simulink model "torqueBalancingYoga2017a"  (Simulink 8.9)
settings: Solver=FixedStepDiscrete  StartTime=0.0  StopTime="Config.SIMULATION_TIME "  FixedStep=Config.Ts  RelTol=1e-3  EnableMultiTasking=on
InitFcn:
  | cd(fileparts(which(bdroot)));
  | initTorqueBalancingYoga;
StopFcn:
  | cd(fileparts(which(bdroot)));
  | stopTorqueBalancingYoga;
undefined symbols (not defined in the file or in its folder): bVectorConstraints, Config, ConstraintsMatrix, Gain, Reg, ROBOT_DOF, ROBOT_DOF_FOR_SIMULINK, Sat, Sm
libraries: WBToolboxLibrary x86, simulink x4
(part 2 of 2)

== system torqueBalancingYoga2017a/controller_QP/Compute angular momentum integral/Compute base to fixed link transform ==
  qj : Inport
  inertial : Inport  Port=2
  Constant7 : Constant  Value=eye(4)
  "LFoot to base link transform " : Subsystem
  LFoot to world transform (fixed base) : WBToolboxLibrary/wholeBodyModel/Kinematics/Forward Kinematics  frameName=Frames.LEFT_FOOT
      settings: SourceProductName=Whole Body Toolbox
  RFoot to base link transform : Subsystem
  RFoot to world transform (fixed base) : WBToolboxLibrary/wholeBodyModel/Kinematics/Forward Kinematics  frameName=Frames.RIGHT_FOOT
      settings: SourceProductName=Whole Body Toolbox
  fixed_LFoot_H_b : Outport
  fixed_RFoot_H_b : Outport  Port=2
  wires:
  Constant7/1 -> RFoot to base link transform/4(w_H_base_fixed), "LFoot to base link transform "/4(w_H_base_fixed), RFoot to world transform (fixed base)/1, LFoot to world transform (fixed base)/1
  RFoot to base link transform/1(link_H_b) -> fixed_RFoot_H_b/1
  "LFoot to base link transform "/1(link_H_b) -> fixed_LFoot_H_b/1
  LFoot to world transform (fixed base)/1 -> "LFoot to base link transform "/3(w_H_link)
  RFoot to world transform (fixed base)/1 -> RFoot to base link transform/3(w_H_link)
  qj/1 -> "LFoot to base link transform "/1(qj), RFoot to base link transform/1(qj), RFoot to world transform (fixed base)/2, LFoot to world transform (fixed base)/2
  inertial/1 -> "LFoot to base link transform "/2(inertial), RFoot to base link transform/2(inertial)

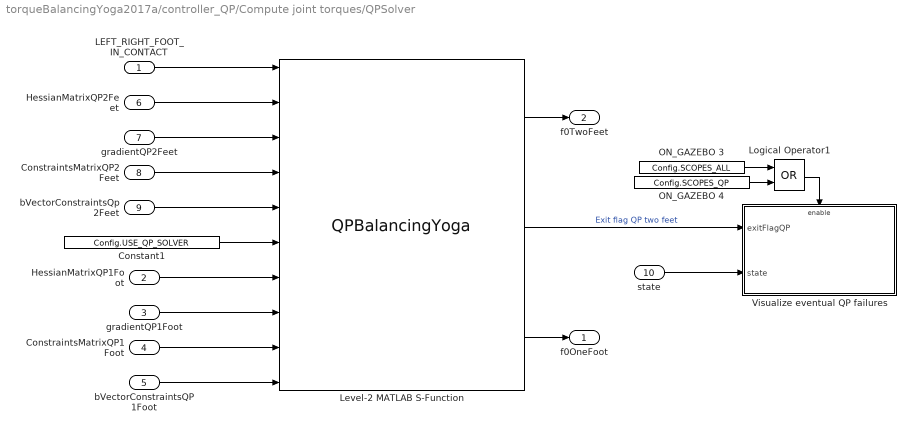
== system torqueBalancingYoga2017a/controller_QP/Compute joint torques/QPSolver ==
  LEFT_RIGHT_FOOT_IN_CONTACT : Inport
  HessianMatrixQP1Foot : Inport  Port=2
  gradientQP1Foot : Inport  Port=3
  ConstraintsMatrixQP1Foot : Inport  Port=4
  bVectorConstraintsQP1Foot : Inport  Port=5
  HessianMatrixQP2Feet : Inport  Port=6
  gradientQP2Feet : Inport  Port=7
  ConstraintsMatrixQP2Feet : Inport  Port=8
  bVectorConstraintsQp2Feet : Inport  Port=9
  state : Inport  Port=10
  Constant1 : Constant  Value=Config.USE_QP_SOLVER
  Level-2 MATLAB S-Function : M-S-Function  FunctionName=QPBalancingYoga
  Logical Operator1 : Logic  Operator=OR  AllPortsSameDT=off  OutDataTypeStr=boolean
  ON_GAZEBO 3 : Constant  Value=Config.SCOPES_ALL
  ON_GAZEBO 4 : Constant  Value=Config.SCOPES_QP
  Visualize eventual QP failures : Subsystem
  f0OneFoot : Outport
  f0TwoFeet : Outport  Port=2
  wires:
  Level-2 MATLAB S-Function/1 -> f0TwoFeet/1
  Level-2 MATLAB S-Function/2 -> Visualize eventual QP failures/1(exitFlagQP)  "Exit flag QP two feet"
  HessianMatrixQP1Foot/1 -> Level-2 MATLAB S-Function/7
  gradientQP1Foot/1 -> Level-2 MATLAB S-Function/8
  ConstraintsMatrixQP1Foot/1 -> Level-2 MATLAB S-Function/9
  bVectorConstraintsQP1Foot/1 -> Level-2 MATLAB S-Function/10
  Level-2 MATLAB S-Function/3 -> f0OneFoot/1
  Logical Operator1/1 -> Visualize eventual QP failures/Enable
  state/1 -> Visualize eventual QP failures/2(state)
  LEFT_RIGHT_FOOT_IN_CONTACT/1 -> Level-2 MATLAB S-Function/1
  HessianMatrixQP2Feet/1 -> Level-2 MATLAB S-Function/2
  gradientQP2Feet/1 -> Level-2 MATLAB S-Function/3
  ConstraintsMatrixQP2Feet/1 -> Level-2 MATLAB S-Function/4
  bVectorConstraintsQp2Feet/1 -> Level-2 MATLAB S-Function/5
  Constant1/1 -> Level-2 MATLAB S-Function/6
  ON_GAZEBO 3/1 -> Logical Operator1/1
  ON_GAZEBO 4/1 -> Logical Operator1/2

== system torqueBalancingYoga2017a/Robot State and References/Internal Coordinator/Base to fixed_link/LFoot to base link transform  ==
  qj : Inport
  inertial : Inport  Port=2
  w_H_link : Inport  Port=3
  w_H_base_fixed : Inport  Port=4
  Fixed base to imu transform : WBToolboxLibrary/wholeBodyModel/Kinematics/Forward Kinematics  frameName=Frames.IMU
      settings: SourceProductName=Whole Body Toolbox
  Fixed base to root link transform : WBToolboxLibrary/wholeBodyModel/Kinematics/Forward Kinematics  frameName=Frames.BASE
      settings: SourceProductName=Whole Body Toolbox
  Inv\* : Product  Inputs=/*  Multiplication=Matrix(*)
  "Inv\\*  " : Product  Inputs=/*  Multiplication=Matrix(*)
  Neck Position : WBToolboxLibrary/Utilities/Yarp Read  portName=Ports.NECK_POS  signalSize=6  timeout=0.5  blocking=off  timestamp=off  autoconnect=on  errorOnConnection=off
      settings: SourceProductName=Whole Body Toolbox
  Switch6 : Switch  Criteria=u2 > Threshold
  USE_IMU4EST_BASE : Constant  Value=Config.USE_IMU4EST_BASE
  fromImuToHomogeousTransformFCN : MATLAB Function  TreatAsAtomicUnit=on
  holder 1 : WBToolboxLibrary/Utilities/holder 
      settings: SourceProductName=Whole Body Toolbox
  holder 2 : WBToolboxLibrary/Utilities/holder 
      settings: SourceProductName=Whole Body Toolbox
  neck transform : Subsystem
  link_H_b : Outport
  wires:
  Switch6/1 -> link_H_b/1
  "Inv\\*  "/1 -> Switch6/3, fromImuToHomogeousTransformFCN/3(link_H_base)  "link_H_root"
  USE_IMU4EST_BASE/1 -> Switch6/2
  Inv\*/1 -> fromImuToHomogeousTransformFCN/1(imu_H_link), holder 1/1  "imu_H_link"
  holder 2/1 -> fromImuToHomogeousTransformFCN/4(inertial_0)
  Fixed base to imu transform/1 -> Inv\*/1
  holder 1/1 -> fromImuToHomogeousTransformFCN/2(imu_H_link_0)
  qj/1 -> Fixed base to imu transform/2, Fixed base to root link transform/2
  fromImuToHomogeousTransformFCN/1(w_H_b) -> Switch6/1
  Fixed base to root link transform/1 -> "Inv\\*  "/2
  inertial/1 -> holder 2/1, fromImuToHomogeousTransformFCN/5(inertial)
  Neck Position/1 -> neck transform/1(neck port)
  neck transform/1(neck position) -> fromImuToHomogeousTransformFCN/6(neck_pos)
  w_H_link/1 -> "Inv\\*  "/1, Inv\*/2
  w_H_base_fixed/1 -> Fixed base to root link transform/1, Fixed base to imu transform/1

== system torqueBalancingYoga2017a/Robot State and References/Internal Coordinator/Compute State Velocity/Feet Jacobians ==
  qj : Inport
  w_H_b : Inport  Port=2
  Jacobian LFoot : WBToolboxLibrary/wholeBodyModel/Jacobians/Jacobian  frameName=Frames.LEFT_FOOT
      settings: SourceProductName=Whole Body Toolbox
  Jacobian RFoot : WBToolboxLibrary/wholeBodyModel/Jacobians/Jacobian  frameName=Frames.RIGHT_FOOT
      settings: SourceProductName=Whole Body Toolbox
  J_LFoot : Outport
  J_RFoot : Outport  Port=2
  wires:
  Jacobian LFoot/1 -> J_LFoot/1
  Jacobian RFoot/1 -> J_RFoot/1
  w_H_b/1 -> Jacobian RFoot/1, Jacobian LFoot/1
  qj/1 -> Jacobian LFoot/2, Jacobian RFoot/2

== system torqueBalancingYoga2017a/Robot State and References/State Machine Yoga/Compute State Velocity/Feet Jacobians ==
  qj : Inport
  w_H_b : Inport  Port=2
  Jacobian LFoot : WBToolboxLibrary/wholeBodyModel/Jacobians/Jacobian  frameName=Frames.LEFT_FOOT
      settings: SourceProductName=Whole Body Toolbox
  Jacobian RFoot : WBToolboxLibrary/wholeBodyModel/Jacobians/Jacobian  frameName=Frames.RIGHT_FOOT
      settings: SourceProductName=Whole Body Toolbox
  J_LFoot : Outport
  J_RFoot : Outport  Port=2
  wires:
  Jacobian LFoot/1 -> J_LFoot/1
  Jacobian RFoot/1 -> J_RFoot/1
  w_H_b/1 -> Jacobian RFoot/1, Jacobian LFoot/1
  qj/1 -> Jacobian LFoot/2, Jacobian RFoot/2

== system torqueBalancingYoga2017a/Robot State and References/State Machine Yoga/Compute base to fixed link transform/LFoot to base link transform  ==
  qj : Inport
  inertial : Inport  Port=2
  w_H_link : Inport  Port=3
  w_H_base_fixed : Inport  Port=4
  Fixed base to imu transform : WBToolboxLibrary/wholeBodyModel/Kinematics/Forward Kinematics  frameName=Frames.IMU
      settings: SourceProductName=Whole Body Toolbox
  Fixed base to root link transform : WBToolboxLibrary/wholeBodyModel/Kinematics/Forward Kinematics  frameName=Frames.BASE
      settings: SourceProductName=Whole Body Toolbox
  Inv\* : Product  Inputs=/*  Multiplication=Matrix(*)
  "Inv\\*  " : Product  Inputs=/*  Multiplication=Matrix(*)
  Neck Position : WBToolboxLibrary/Utilities/Yarp Read  portName=Ports.NECK_POS  signalSize=6  timeout=0.5  blocking=off  timestamp=off  autoconnect=on  errorOnConnection=off
      settings: SourceProductName=Whole Body Toolbox
  Switch6 : Switch  Criteria=u2 > Threshold
  USE_IMU4EST_BASE : Constant  Value=Config.USE_IMU4EST_BASE
  fromImuToHomogeousTransformFCN : MATLAB Function  TreatAsAtomicUnit=on
  holder 1 : WBToolboxLibrary/Utilities/holder 
      settings: SourceProductName=Whole Body Toolbox
  holder 2 : WBToolboxLibrary/Utilities/holder 
      settings: SourceProductName=Whole Body Toolbox
  neck transform : Subsystem
  link_H_b : Outport
  wires:
  Switch6/1 -> link_H_b/1
  "Inv\\*  "/1 -> Switch6/3, fromImuToHomogeousTransformFCN/3(link_H_base)  "link_H_root"
  USE_IMU4EST_BASE/1 -> Switch6/2
  Inv\*/1 -> fromImuToHomogeousTransformFCN/1(imu_H_link), holder 1/1  "imu_H_link"
  holder 2/1 -> fromImuToHomogeousTransformFCN/4(inertial_0)
  Fixed base to imu transform/1 -> Inv\*/1
  holder 1/1 -> fromImuToHomogeousTransformFCN/2(imu_H_link_0)
  qj/1 -> Fixed base to imu transform/2, Fixed base to root link transform/2
  fromImuToHomogeousTransformFCN/1(w_H_b) -> Switch6/1
  Fixed base to root link transform/1 -> "Inv\\*  "/2
  inertial/1 -> holder 2/1, fromImuToHomogeousTransformFCN/5(inertial)
  Neck Position/1 -> neck transform/1(neck port)
  neck transform/1(neck position) -> fromImuToHomogeousTransformFCN/6(neck_pos)
  w_H_link/1 -> "Inv\\*  "/1, Inv\*/2
  w_H_base_fixed/1 -> Fixed base to root link transform/1, Fixed base to imu transform/1

== system torqueBalancingYoga2017a/Robot State and References/State Machine Yoga/Compute base to fixed link transform/RFoot to base link transform ==
  qj : Inport
  inertial : Inport  Port=2
  w_H_link : Inport  Port=3
  w_H_base_fixed : Inport  Port=4
  Fixed base to imu transform : WBToolboxLibrary/wholeBodyModel/Kinematics/Forward Kinematics  frameName=Frames.IMU
      settings: SourceProductName=Whole Body Toolbox
  Fixed base to root link transform : WBToolboxLibrary/wholeBodyModel/Kinematics/Forward Kinematics  frameName=Frames.BASE
      settings: SourceProductName=Whole Body Toolbox
  Inv\* : Product  Inputs=/*  Multiplication=Matrix(*)
  "Inv\\*  " : Product  Inputs=/*  Multiplication=Matrix(*)
  Neck Position : WBToolboxLibrary/Utilities/Yarp Read  portName=Ports.NECK_POS  signalSize=6  timeout=0.5  blocking=off  timestamp=off  autoconnect=on  errorOnConnection=off
      settings: SourceProductName=Whole Body Toolbox
  Switch6 : Switch  Criteria=u2 > Threshold
  USE_IMU4EST_BASE : Constant  Value=Config.USE_IMU4EST_BASE
  fromImuToHomogeousTransformFCN : MATLAB Function  TreatAsAtomicUnit=on
  holder 1 : WBToolboxLibrary/Utilities/holder 
      settings: SourceProductName=Whole Body Toolbox
  holder 2 : WBToolboxLibrary/Utilities/holder 
      settings: SourceProductName=Whole Body Toolbox
  neck transform : Subsystem
  link_H_b : Outport
  wires:
  Switch6/1 -> link_H_b/1
  "Inv\\*  "/1 -> Switch6/3, fromImuToHomogeousTransformFCN/3(link_H_base)  "link_H_root"
  USE_IMU4EST_BASE/1 -> Switch6/2
  Inv\*/1 -> fromImuToHomogeousTransformFCN/1(imu_H_link), holder 1/1  "imu_H_link"
  holder 2/1 -> fromImuToHomogeousTransformFCN/4(inertial_0)
  Fixed base to imu transform/1 -> Inv\*/1
  holder 1/1 -> fromImuToHomogeousTransformFCN/2(imu_H_link_0)
  qj/1 -> Fixed base to imu transform/2, Fixed base to root link transform/2
  fromImuToHomogeousTransformFCN/1(w_H_b) -> Switch6/1
  Fixed base to root link transform/1 -> "Inv\\*  "/2
  inertial/1 -> holder 2/1, fromImuToHomogeousTransformFCN/5(inertial)
  Neck Position/1 -> neck transform/1(neck port)
  neck transform/1(neck position) -> fromImuToHomogeousTransformFCN/6(neck_pos)
  w_H_link/1 -> "Inv\\*  "/1, Inv\*/2
  w_H_base_fixed/1 -> Fixed base to root link transform/1, Fixed base to imu transform/1

== system torqueBalancingYoga2017a/controller_QP/Compute angular momentum integral/Compute base to fixed link transform/LFoot to base link transform  ==
  qj : Inport
  inertial : Inport  Port=2
  w_H_link : Inport  Port=3
  w_H_base_fixed : Inport  Port=4
  Fixed base to imu transform : WBToolboxLibrary/wholeBodyModel/Kinematics/Forward Kinematics  frameName=Frames.IMU
      settings: SourceProductName=Whole Body Toolbox
  Fixed base to root link transform : WBToolboxLibrary/wholeBodyModel/Kinematics/Forward Kinematics  frameName=Frames.BASE
      settings: SourceProductName=Whole Body Toolbox
  Inv\* : Product  Inputs=/*  Multiplication=Matrix(*)
  "Inv\\*  " : Product  Inputs=/*  Multiplication=Matrix(*)
  Neck Position : WBToolboxLibrary/Utilities/Yarp Read  portName=Ports.NECK_POS  signalSize=6  timeout=0.5  blocking=off  timestamp=off  autoconnect=on  errorOnConnection=off
      settings: SourceProductName=Whole Body Toolbox
  Switch6 : Switch  Criteria=u2 > Threshold
  USE_IMU4EST_BASE : Constant  Value=Config.USE_IMU4EST_BASE
  fromImuToHomogeousTransformFCN : MATLAB Function  TreatAsAtomicUnit=on
  holder 1 : WBToolboxLibrary/Utilities/holder 
      settings: SourceProductName=Whole Body Toolbox
  holder 2 : WBToolboxLibrary/Utilities/holder 
      settings: SourceProductName=Whole Body Toolbox
  neck transform : Subsystem
  link_H_b : Outport
  wires:
  Switch6/1 -> link_H_b/1
  "Inv\\*  "/1 -> Switch6/3, fromImuToHomogeousTransformFCN/3(link_H_base)  "link_H_root"
  USE_IMU4EST_BASE/1 -> Switch6/2
  Inv\*/1 -> fromImuToHomogeousTransformFCN/1(imu_H_link), holder 1/1  "imu_H_link"
  holder 2/1 -> fromImuToHomogeousTransformFCN/4(inertial_0)
  Fixed base to imu transform/1 -> Inv\*/1
  holder 1/1 -> fromImuToHomogeousTransformFCN/2(imu_H_link_0)
  qj/1 -> Fixed base to imu transform/2, Fixed base to root link transform/2
  fromImuToHomogeousTransformFCN/1(w_H_b) -> Switch6/1
  Fixed base to root link transform/1 -> "Inv\\*  "/2
  inertial/1 -> holder 2/1, fromImuToHomogeousTransformFCN/5(inertial)
  Neck Position/1 -> neck transform/1(neck port)
  neck transform/1(neck position) -> fromImuToHomogeousTransformFCN/6(neck_pos)
  w_H_link/1 -> "Inv\\*  "/1, Inv\*/2
  w_H_base_fixed/1 -> Fixed base to root link transform/1, Fixed base to imu transform/1

== system torqueBalancingYoga2017a/controller_QP/Compute angular momentum integral/Compute base to fixed link transform/RFoot to base link transform ==
  qj : Inport
  inertial : Inport  Port=2
  w_H_link : Inport  Port=3
  w_H_base_fixed : Inport  Port=4
  Fixed base to imu transform : WBToolboxLibrary/wholeBodyModel/Kinematics/Forward Kinematics  frameName=Frames.IMU
      settings: SourceProductName=Whole Body Toolbox
  Fixed base to root link transform : WBToolboxLibrary/wholeBodyModel/Kinematics/Forward Kinematics  frameName=Frames.BASE
      settings: SourceProductName=Whole Body Toolbox
  Inv\* : Product  Inputs=/*  Multiplication=Matrix(*)
  "Inv\\*  " : Product  Inputs=/*  Multiplication=Matrix(*)
  Neck Position : WBToolboxLibrary/Utilities/Yarp Read  portName=Ports.NECK_POS  signalSize=6  timeout=0.5  blocking=off  timestamp=off  autoconnect=on  errorOnConnection=off
      settings: SourceProductName=Whole Body Toolbox
  Switch6 : Switch  Criteria=u2 > Threshold
  USE_IMU4EST_BASE : Constant  Value=Config.USE_IMU4EST_BASE
  fromImuToHomogeousTransformFCN : MATLAB Function  TreatAsAtomicUnit=on
  holder 1 : WBToolboxLibrary/Utilities/holder 
      settings: SourceProductName=Whole Body Toolbox
  holder 2 : WBToolboxLibrary/Utilities/holder 
      settings: SourceProductName=Whole Body Toolbox
  neck transform : Subsystem
  link_H_b : Outport
  wires:
  Switch6/1 -> link_H_b/1
  "Inv\\*  "/1 -> Switch6/3, fromImuToHomogeousTransformFCN/3(link_H_base)  "link_H_root"
  USE_IMU4EST_BASE/1 -> Switch6/2
  Inv\*/1 -> fromImuToHomogeousTransformFCN/1(imu_H_link), holder 1/1  "imu_H_link"
  holder 2/1 -> fromImuToHomogeousTransformFCN/4(inertial_0)
  Fixed base to imu transform/1 -> Inv\*/1
  holder 1/1 -> fromImuToHomogeousTransformFCN/2(imu_H_link_0)
  qj/1 -> Fixed base to imu transform/2, Fixed base to root link transform/2
  fromImuToHomogeousTransformFCN/1(w_H_b) -> Switch6/1
  Fixed base to root link transform/1 -> "Inv\\*  "/2
  inertial/1 -> holder 2/1, fromImuToHomogeousTransformFCN/5(inertial)
  Neck Position/1 -> neck transform/1(neck port)
  neck transform/1(neck position) -> fromImuToHomogeousTransformFCN/6(neck_pos)
  w_H_link/1 -> "Inv\\*  "/1, Inv\*/2
  w_H_base_fixed/1 -> Fixed base to root link transform/1, Fixed base to imu transform/1

== system torqueBalancingYoga2017a/controller_QP/Compute joint torques/QPSolver/Visualize eventual QP failures ==
  exitFlagQP : Inport
  state : Inport  Port=2
  Enable : EnablePort
  "QP status (0: no failure, 1: not using)" : Scope  NumInputPorts=2
  wires:
  exitFlagQP/1 -> "QP status (0: no failure, 1: not using)"/1  "exitFlagQP"
  state/1 -> "QP status (0: no failure, 1: not using)"/2

== system torqueBalancingYoga2017a/Robot State and References/Internal Coordinator/Base to fixed_link/LFoot to base link transform /neck transform ==
  neck port : Inport
  Constant : Constant  Value=zeros(3,1)
  Gain : Gain  Gain=pi/180
  Selector1 : Selector  InputPortWidth=6  IndexOptions=Index vector (dialog)  Indices=[1:3]  OutputSizes=1
  Switch : Switch  Criteria=u2 > Threshold
  USE_IMU4EST_BASE1 : Constant  Value=Config.CORRECT_NECK_IMU
  neck position : Outport
  wires:
  neck port/1 -> Gain/1
  USE_IMU4EST_BASE1/1 -> Switch/2
  Switch/1 -> neck position/1
  Gain/1 -> Selector1/1
  Constant/1 -> Switch/3
  Selector1/1 -> Switch/1  "neck pos"

== system torqueBalancingYoga2017a/Robot State and References/State Machine Yoga/Compute base to fixed link transform/LFoot to base link transform /neck transform ==
  neck port : Inport
  Constant : Constant  Value=zeros(3,1)
  Gain : Gain  Gain=pi/180
  Selector1 : Selector  InputPortWidth=6  IndexOptions=Index vector (dialog)  Indices=[1:3]  OutputSizes=1
  Switch : Switch  Criteria=u2 > Threshold
  USE_IMU4EST_BASE1 : Constant  Value=Config.CORRECT_NECK_IMU
  neck position : Outport
  wires:
  neck port/1 -> Gain/1
  USE_IMU4EST_BASE1/1 -> Switch/2
  Switch/1 -> neck position/1
  Gain/1 -> Selector1/1
  Constant/1 -> Switch/3
  Selector1/1 -> Switch/1  "neck pos"

== system torqueBalancingYoga2017a/Robot State and References/State Machine Yoga/Compute base to fixed link transform/RFoot to base link transform/neck transform ==
  neck port : Inport
  Constant : Constant  Value=zeros(3,1)
  Gain : Gain  Gain=pi/180
  Selector1 : Selector  InputPortWidth=6  IndexOptions=Index vector (dialog)  Indices=[1:3]  OutputSizes=1
  Switch : Switch  Criteria=u2 > Threshold
  USE_IMU4EST_BASE1 : Constant  Value=Config.CORRECT_NECK_IMU
  neck position : Outport
  wires:
  neck port/1 -> Gain/1
  USE_IMU4EST_BASE1/1 -> Switch/2
  Switch/1 -> neck position/1
  Gain/1 -> Selector1/1
  Constant/1 -> Switch/3
  Selector1/1 -> Switch/1  "neck pos"

== system torqueBalancingYoga2017a/controller_QP/Compute angular momentum integral/Compute base to fixed link transform/LFoot to base link transform /neck transform ==
  neck port : Inport
  Constant : Constant  Value=zeros(3,1)
  Gain : Gain  Gain=pi/180
  Selector1 : Selector  InputPortWidth=6  IndexOptions=Index vector (dialog)  Indices=[1:3]  OutputSizes=1
  Switch : Switch  Criteria=u2 > Threshold
  USE_IMU4EST_BASE1 : Constant  Value=Config.CORRECT_NECK_IMU
  neck position : Outport
  wires:
  neck port/1 -> Gain/1
  USE_IMU4EST_BASE1/1 -> Switch/2
  Switch/1 -> neck position/1
  Gain/1 -> Selector1/1
  Constant/1 -> Switch/3
  Selector1/1 -> Switch/1  "neck pos"

== system torqueBalancingYoga2017a/controller_QP/Compute angular momentum integral/Compute base to fixed link transform/RFoot to base link transform/neck transform ==
  neck port : Inport
  Constant : Constant  Value=zeros(3,1)
  Gain : Gain  Gain=pi/180
  Selector1 : Selector  InputPortWidth=6  IndexOptions=Index vector (dialog)  Indices=[1:3]  OutputSizes=1
  Switch : Switch  Criteria=u2 > Threshold
  USE_IMU4EST_BASE1 : Constant  Value=Config.CORRECT_NECK_IMU
  neck position : Outport
  wires:
  neck port/1 -> Gain/1
  USE_IMU4EST_BASE1/1 -> Switch/2
  Switch/1 -> neck position/1
  Gain/1 -> Selector1/1
  Constant/1 -> Switch/3
  Selector1/1 -> Switch/1  "neck pos"

== matlab function controller_QP/Compute angular momentum integral/Compute base to fixed link transform/LFoot to base link transform /fromImuToHomogeousTransformFCN ==
  data: imu_H_link input double; imu_H_link_0 input double; link_H_base input double; inertial_0 input double; inertial input double; neck_pos input double; w_H_b output double; Config parameter double
function w_H_b = worldToBaseTransformWithIMUFCN(imu_H_link,imu_H_link_0,link_H_base,inertial_0,inertial,neck_pos,Config)

    w_H_b = worldToBaseTransformWithIMU(imu_H_link,imu_H_link_0,link_H_base,inertial_0,inertial,neck_pos,Config);

end

== matlab function Robot State and References/Internal Coordinator/Base to fixed_link/LFoot to base link transform /fromImuToHomogeousTransformFCN ==
  data: imu_H_link input double; imu_H_link_0 input double; link_H_base input double; inertial_0 input double; inertial input double; neck_pos input double; w_H_b output double; Config parameter double
function w_H_b = worldToBaseTransformWithIMUFCN(imu_H_link,imu_H_link_0,link_H_base,inertial_0,inertial,neck_pos,Config)

    w_H_b = worldToBaseTransformWithIMU(imu_H_link,imu_H_link_0,link_H_base,inertial_0,inertial,neck_pos,Config);

end

== matlab function Robot State and References/State Machine Yoga/Compute base to fixed link transform/RFoot to base link transform/fromImuToHomogeousTransformFCN ==
  data: imu_H_link input double; imu_H_link_0 input double; link_H_base input double; inertial_0 input double; inertial input double; neck_pos input double; w_H_b output double; Config parameter double
function w_H_b = worldToBaseTransformWithIMUFCN(imu_H_link,imu_H_link_0,link_H_base,inertial_0,inertial,neck_pos,Config)

    w_H_b = worldToBaseTransformWithIMU(imu_H_link,imu_H_link_0,link_H_base,inertial_0,inertial,neck_pos,Config);

end

== matlab function controller_QP/Compute angular momentum integral/Compute base to fixed link transform/RFoot to base link transform/fromImuToHomogeousTransformFCN ==
  data: imu_H_link input double; imu_H_link_0 input double; link_H_base input double; inertial_0 input double; inertial input double; neck_pos input double; w_H_b output double; Config parameter double
function w_H_b = worldToBaseTransformWithIMUFCN(imu_H_link,imu_H_link_0,link_H_base,inertial_0,inertial,neck_pos,Config)

    w_H_b = worldToBaseTransformWithIMU(imu_H_link,imu_H_link_0,link_H_base,inertial_0,inertial,neck_pos,Config);

end

== matlab function Robot State and References/Internal Coordinator/Compute State Velocity/Compute Base Velocity ==
  data: J_LeftFoot input double; J_RightFoot input double; feetInContact input double; nu_b output double; qjDot input double; Reg parameter double
function nu_b = computeBaseVelocityFCN(J_LeftFoot, J_RightFoot, feetInContact, qjDot, Reg)

    nu_b = computeBaseVelocity(J_LeftFoot, J_RightFoot, feetInContact, qjDot, Reg);
end

== matlab function Dynamics and Kinematics/Dynamics/Add motors reflected inertias/Add motor reflected inertias ==
  data: M input double; M_with_inertia output double; Config parameter double
function M_with_inertia = addMotorsInertiaFCN(M,Config)

    M_with_inertia = addMotorsInertia(M,Config);

end

== matlab function Robot State and References/State Machine Yoga/Compute State Velocity/Compute Base Velocity ==
  data: J_LeftFoot input double; J_RightFoot input double; feetInContact input double; nu_b output double; qjDot input double; Reg parameter double
function nu_b = computeBaseVelocityFCN(J_LeftFoot, J_RightFoot, feetInContact, qjDot, Reg)

    nu_b = computeBaseVelocity(J_LeftFoot, J_RightFoot, feetInContact, qjDot, Reg);
end

== matlab function Robot State and References/State Machine Yoga/Compute base to fixed link transform/LFoot to base link transform /fromImuToHomogeousTransformFCN ==
  data: imu_H_link input double; imu_H_link_0 input double; link_H_base input double; inertial_0 input double; inertial input double; neck_pos input double; w_H_b output double; Config parameter double
function w_H_b = worldToBaseTransformWithIMUFCN(imu_H_link,imu_H_link_0,link_H_base,inertial_0,inertial,neck_pos,Config)

    w_H_b = worldToBaseTransformWithIMU(imu_H_link,imu_H_link_0,link_H_base,inertial_0,inertial,neck_pos,Config);

end

== matlab function controller_QP/Compute joint torques (motor reflected inertia)/(transpose(T*Gamma))^{-1}*I_m*(T*Gamma)^{-1} ==
  data: reflectedInertia output double; Config parameter double
function reflectedInertia  = computeMotorsInertiaFCN(Config)

    [reflectedInertia] = computeMotorsInertia(Config);

end

== matlab function Robot State and References/Internal Coordinator/Reference Generator CoM ==
  data: pos_CoM_0 input double; t input double; references_CoM output double; Config parameter double
function references_CoM = referenceGeneratorCoMFCN(pos_CoM_0, t, Config)

    references_CoM = referenceGeneratorCoM(pos_CoM_0, t, Config);
end

== matlab function tauDot Saturation/Saturate the Torque Derivative ==
  data: u input double; uSat output double; u_0 input double; Config parameter double
function uSat = saturateInputDerivativeFCN(u, u_0, Config)

    uSat = saturateInputDerivative(u, u_0, Config);

end

== matlab function Robot State and References/State Machine Yoga/stateMachineYogaFCN ==
  data: wrench_rightFoot input double; wrench_leftFoot input double; w_H_b output double; CoM_des output double; qj_des output double; constraints output double; CoM_0 input double; q0 input double; l_sole_CoM input double; r_sole_CoM input double; qj input double; t input double; l_sole_H_b input double; r_sole_H_b input double; Sm parameter double; impedances output double; KPCoM output double; KDCoM output double; Gain parameter double; currentState output double; jointsSmoothingTime output double
function [w_H_b, CoM_des, qj_des, constraints, impedances, KPCoM, KDCoM, currentState, jointsSmoothingTime] = ...
          stateMachineYogaFCN(wrench_rightFoot, wrench_leftFoot, CoM_0, q0, l_sole_CoM, r_sole_CoM, qj, t, l_sole_H_b, r_sole_H_b, Sm, Gain)
 
    [w_H_b, CoM_des, qj_des, constraints, impedances, KPCoM, KDCoM, currentState, jointsSmoothingTime] = ...
        stateMachineYoga(CoM_0, q0, l_sole_CoM, r_sole_CoM, qj, t, wrench_rightFoot, wrench_leftFoot, l_sole_H_b, r_sole_H_b, Sm, Gain); 
end

== matlab function controller_QP/Balancing Controller  ==
  data: tauModel output double; Sigma output double; NA output double; fHdotDesC1C2 output double; HessianMatrixQP1Foot output double; gradientQP1Foot output double; ConstraintsMatrixQP1Foot output double; bVectorConstraintsQp1Foot output double; HessianMatrixQP2Feet output double; gradientQP2Feet output double; ConstraintsMatrixQP2Feet output double; bVectorConstraintsQp2Feet output double; constraints input double; ROBOT_DOF_FOR_SIMULINK input double; ConstraintsMatrix input double; bVectorConstraints input double; qj input double; qjDes input double; nu input double; M input double; h input double; H input double; intHw input double; w_H_l_sole input double; w_H_r_sole input double; JL input double; JR input double; dJLv input double; dJRv input double; xCoM input double; J_CoM input double; desired_x_dx_ddx_CoM input double; gainsPCOM input double; gainsDCOM input double; impedances input double; errorCoM output double; f_noQP output double; Gain parameter double; Reg parameter double
function [tauModel, Sigma, NA, fHdotDesC1C2, ...
          HessianMatrixQP1Foot, gradientQP1Foot, ConstraintsMatrixQP1Foot, bVectorConstraintsQp1Foot, ...
          HessianMatrixQP2Feet, gradientQP2Feet, ConstraintsMatrixQP2Feet, bVectorConstraintsQp2Feet, ...
          errorCoM,f_noQP] = ...
              balancingControllerYogaFCN(constraints, ROBOT_DOF_FOR_SIMULINK, ConstraintsMatrix, bVectorConstraints, ...
                  qj, qjDes, nu, M, h, H, intHw, w_H_l_sole, w_H_r_sole, JL, JR, dJLv, dJRv, xCoM, J_CoM, desired_x_dx_ddx_CoM, ...
                  gainsPCOM, gainsDCOM, impedances, Gain, Reg)
          
    [tauModel, Sigma, NA, fHdotDesC1C2, ...
     HessianMatrixQP1Foot, gradientQP1Foot, ConstraintsMatrixQP1Foot, bVectorConstraintsQp1Foot, ...
     HessianMatrixQP2Feet, gradientQP2Feet, ConstraintsMatrixQP2Feet, bVectorConstraintsQp2Feet, ...
     errorCoM, f_noQP] = ...
         balancingControllerYoga(constraints, ROBOT_DOF_FOR_SIMULINK, ConstraintsMatrix, bVectorConstraints, ...
                                 qj, qjDes, nu, M, h, H, intHw, w_H_l_sole, w_H_r_sole, JL, JR, dJLv, dJRv, xCoM, J_CoM, desired_x_dx_ddx_CoM, ...
                                 gainsPCOM, gainsDCOM, impedances, Reg, Gain);
end

== matlab function emergency stop: joint limits/MATLAB Function ==
  data: umin input double; umax input double; u input double; inRange output double; tol input double
function inRange = checkRangeFCN(umin, umax, u, tol)

     inRange = checkRange(umin, umax, u, tol);
end

== matlab function controller_QP/Compute angular momentum integral/choose base to world transform ==
  data: state input double; booleanState output double
function booleanState = footOnGround(state)

    % output: a boolean variable whose value is 1 if the foot on ground is left
    % foot, and 0 if the foot on ground is the right foot. If both feet are on
    % ground, the variable is setted to 1.

    % states in which right foot is on ground: 9,10,11,12
    booleanState = 1;

    if state == 9 || state == 10 || state == 11 || state == 12

        booleanState = 0;
    end
end

== matlab function controller_QP/Compute angular momentum integral/References for H ==
  data: qjErr input double; JL input double; JR input double; nu_b_equivalent output double; Reg parameter double; activeFeetConstraints input double
function nu_b_equivalent = generateReferencesForH_FCN(qjErr, JL, JR, Reg, activeFeetConstraints)

    if activeFeetConstraints(1) == 1
    
        pinvJb          = (JL(:,1:6)'*JL(:,1:6) + Reg.pinvDamp_nu_b*eye(6))\JL(:,1:6)';
        nu_b_equivalent = -pinvJb*JL(:,7:end)*qjErr;
    else
    
        pinvJb          = (JR(:,1:6)'*JR(:,1:6) + Reg.pinvDamp_nu_b*eye(6))\JR(:,1:6)';
        nu_b_equivalent = -pinvJb*JR(:,7:end)*qjErr;
    end
end
